simulink model "basicModelWithMonod"  (R2024b)
settings: Solver=VariableStepAuto  StartTime=0.0  StopTime=10.0  RelTol=1e-3
values from neighbouring files (symbols this model uses):
  D = 0.1    [TP1_Entregable.m]
  F = zeros(4,1)    [TP1_Entregable.m]
  Q = zeros(4,1)    [TP1_Entregable.m]
  xi0 = [x0;s0;n0;p0]    [TP1_Entregable.m]
  xi_in = [0,0; s_in,0; 0,n_in; 0,0]    [TP1_Entregable.m]
settings Model: Creator=tomii  LastModifiedBy=tomi

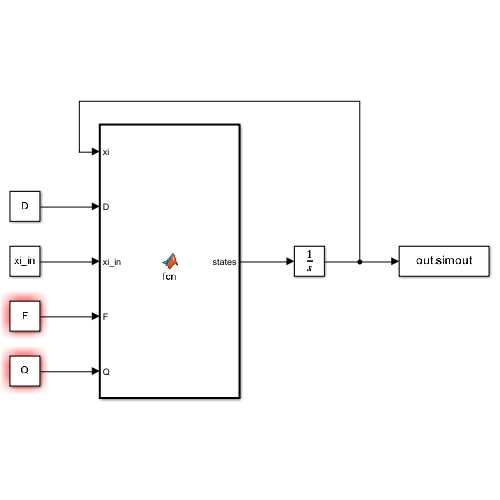
[thumbnail: Simulink's stored preview of the top-level diagram]
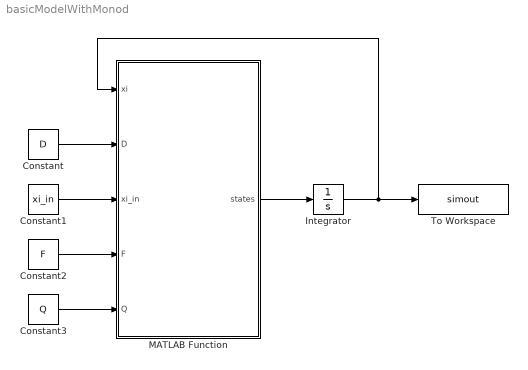
== system basicModelWithMonod ==
  Constant : Constant  Value=D
  Constant1 : Constant  Value=xi_in
  Constant2 : Constant  Value=F
  Constant3 : Constant  Value=Q
  Integrator : Integrator  InitialCondition=xi0
  MATLAB Function : MATLAB Function  TreatAsAtomicUnit=on
  To Workspace : ToWorkspace  VariableName=simout  SaveFormat=Timeseries  SampleTime=-1
  wires:
  MATLAB Function/1(states) -> Integrator/1
  Integrator/1 -> To Workspace/1, MATLAB Function/1(xi)
  Constant/1 -> MATLAB Function/2(D)
  Constant1/1 -> MATLAB Function/3(xi_in)
  Constant2/1 -> MATLAB Function/4(F)
  Constant3/1 -> MATLAB Function/5(Q)

== matlab function basicModelWithMonod/MATLAB Function ==
  data: states output; xi input; D input; xi_in input; F input; Q input; modelParameters parameter
function states = fcn(xi, D, xi_in, F, Q, modelParameters)

% Estados
x=xi(1);
s=xi(2);
n=xi(3);
c=xi(4);

% Modelo de Monod
mumax=modelParameters.mumax;
Ks=modelParameters.Ks;
K=modelParameters.K;

r=mumax*x*(s/(s+Ks));

states = K * r + D * xi_in - D * xi + F - Q;
